simulink model "ADIA"  (R2018b)
settings: Solver=FixedStepDiscrete  StartTime=0.0  StopTime=10.0  FixedStep=0.02  RelTol=1e-3
undefined symbols (not defined in the file or in its folder): ACC_State_Active, ACC_State_BrakeOnly, ACC_State_Suspended, ACC_State_WaitingRise, ADAS_AEBBrakingProg, ADAS_DeclControlReq, ADAS_DriveOff, ADAS_ESCHoldReq_NotHold, ADASDecType_ACC, ADASDecType_AEB, ADIA_ACC_Acceleration_OOR_DecCount_C, ADIA_ACC_Acceleration_OOR_Duration_C, ADIA_ACC_Acceleration_OOR_IncCount_C, ADIA_ACC_Acceleration_OOR_LLim_C, ADIA_ACC_Acceleration_OOR_ULim_C, ADIA_ACC_AccelTrqReq_MixedDia_ULim_C, ADIA_ACC_AccelTrqReq_ULim_C, ADIA_ACC_Deceleration_Mixed_ULim_C, ADIA_ACC_Deceleration_OOR_DecCount_C, ADIA_ACC_Deceleration_OOR_Duration_C, ADIA_ACC_Deceleration_OOR_IncCount_C, ADIA_ACC_Deceleration_OOR_LLim_C, ADIA_ACC_Deceleration_OOR_ULim_C, ADIA_ACC_DriveOff_Distance_C, ADIA_ACC_DriveOff_TimeLim_C, ADIA_ACC_ReqMixed_DecCount_C, ADIA_ACC_ReqMixed_Duration_C, ADIA_ACC_ReqMixed_IncCount_C, ADIA_AccPedalRaw_MaxLim_C, ADIA_AccPedalRaw_MinLim_C, ADIA_ADAS_HoldDecReq_Set_C, ADIA_ADAS_HoldRConfirm_TimeLim_C, ADIA_ADAS_HoldVehSpd_Lim_C, ADIA_AEB_VehSpdDec_LLim_C, ADIA_AEB_VehSpdDec_ULim_C, ADIA_ASWFault_OvrdEn_C, ADIA_ASWFault_OvrdValue_C, ADIA_BatteryOutOfRange_DecCount_C, ADIA_BatteryOutOfRange_Duration_C, ADIA_BatteryOutOfRange_IncCount_C, ADIA_BattVolt_MaxLim_C, ADIA_BattVolt_MinLim_C, ADIA_BCM3_33C_InvBrkLight_DecCount_C, ADIA_BCM3_33C_InvBrkLight_Duration_C, ADIA_BCM3_33C_InvBrkLight_IncCount_C, ADIA_BCM_BattVolt_OvrdEn_C, ADIA_BCM_BattVolt_OvrdVal_C, ADIA_BCM_BrakeLampStaus_OvrdEn_C, ADIA_BCM_BrakeLampStaus_OvrdVal_C, ADIA_BCM_CHMSLStaus_OvrdEn_C, ADIA_BCM_CHMSLStaus_OvrdVal_C, ADIA_BCM_LeftTurnSwSt_OvrdEn_C, ADIA_BCM_LeftTurnSwSt_OvrdVal_C, ADIA_BCM_RightTurnSwSt_OvrdEn_C, ADIA_BCM_RightTurnSwSt_OvrdVal_C, ADIA_BCM_TurnSwFailure_DecCount_C, ADIA_BCM_TurnSwFailure_Duration_C, ADIA_BCM_TurnSwFailure_IncCount_C, ADIA_BSWFault_Ignore_C, ADIA_BSWFault_OvrdEn_C ... (+281)
libraries: simulink x208
(part 10 of 10)

== system ADIA/ADAS_Diagnostics/Diagnostics_Processing/Rationality_Diagnostics/SAS_A5_InvRotSpeed/Counter&Latch/Timer1 ==
  incrcondition : Inport
  incrvalue : Inport  Port=2
  decrcondition : Inport  Port=3
  decvalue : Inport  Port=4
  maxlimit : Inport  Port=5
  reset : Inport  Port=6
  Constant{,1..3} (4 alike) : Constant  Value=0  OutDataTypeStr=Inherit: Inherit via back propagation
  MinMax1 : MinMax  Inputs=2  OutDataTypeStr=Inherit: Inherit via back propagation  InputSameDT=on
  MinMax2 : MinMax  Function=max  Inputs=2  OutDataTypeStr=Inherit: Inherit via back propagation  InputSameDT=on
  Relational Operator : RelationalOperator  OutDataTypeStr=boolean  RndMeth=Nearest
  Sum : Sum  Inputs=++-  OutDataTypeStr=Inherit: Inherit via back propagation  InputSameDT=on
  Unit Delay : UnitDelay  SampleTime=-1
  dec switch : Switch  Criteria=u2 ~= 0  Threshold=1  OutDataTypeStr=Inherit: Inherit via back propagation  InputSameDT=on
  inc switch : Switch  Criteria=u2 ~= 0  Threshold=1  OutDataTypeStr=Inherit: Inherit via back propagation  InputSameDT=on
  reset switch : Switch  Criteria=u2 ~= 0  Threshold=1  OutDataTypeStr=Inherit: Inherit via back propagation  InputSameDT=on
  counter out : Outport
  counter_status : Outport  Port=2
  wires:
  decvalue/1 -> dec switch/1
  Relational Operator/1 -> counter_status/1
  Constant3/1 -> reset switch/1
  inc switch/1 -> Sum/2
  Sum/1 -> MinMax2/2
  maxlimit/1 -> MinMax1/2, Relational Operator/2
  Constant2/1 -> MinMax2/1
  reset switch/1 -> counter out/1, Relational Operator/1, Unit Delay/1
  Unit Delay/1 -> Sum/1
  reset/1 -> reset switch/2
  Constant/1 -> inc switch/3
  MinMax2/1 -> MinMax1/1
  incrvalue/1 -> inc switch/1
  MinMax1/1 -> reset switch/3
  dec switch/1 -> Sum/3
  Constant1/1 -> dec switch/3
  decrcondition/1 -> dec switch/2
  incrcondition/1 -> inc switch/2

== system ADIA/ADAS_Diagnostics/Diagnostics_Processing/Rationality_Diagnostics/SCC_309_OorACCButton/Counter&Latch/Latch  ==
  Input : Inport
  Latch Reset : Inport  Port=2
  Constant11 : Constant  Value=0  OutDataTypeStr=Inherit: Inherit via back propagation
  Constant12 : Constant  OutDataTypeStr=Inherit: Inherit via back propagation
  Switch : Switch  Threshold=1  OutDataTypeStr=Inherit: Inherit via back propagation  SaturateOnIntegerOverflow=on  InputSameDT=on
  Switch1 : Switch  Threshold=1  OutDataTypeStr=Inherit: Inherit via back propagation  SaturateOnIntegerOverflow=on  InputSameDT=on
  Unit Delay1 : UnitDelay  SampleTime=-1
  Output : Outport  InitialOutput=0
  wires:
  Constant12/1 -> Switch1/1
  Constant11/1 -> Switch/1
  Input/1 -> Switch1/2
  Unit Delay1/1 -> Switch1/3
  Switch/1 -> Unit Delay1/1, Output/1
  Latch Reset/1 -> Switch/2
  Switch1/1 -> Switch/3

== system ADIA/ADAS_Diagnostics/Diagnostics_Processing/Rationality_Diagnostics/SCC_309_OorACCButton/Counter&Latch/Timer1 ==
  incrcondition : Inport
  incrvalue : Inport  Port=2
  decrcondition : Inport  Port=3
  decvalue : Inport  Port=4
  maxlimit : Inport  Port=5
  reset : Inport  Port=6
  Constant{,1..3} (4 alike) : Constant  Value=0  OutDataTypeStr=Inherit: Inherit via back propagation
  MinMax1 : MinMax  Inputs=2  OutDataTypeStr=Inherit: Inherit via back propagation  InputSameDT=on
  MinMax2 : MinMax  Function=max  Inputs=2  OutDataTypeStr=Inherit: Inherit via back propagation  InputSameDT=on
  Relational Operator : RelationalOperator  OutDataTypeStr=boolean  RndMeth=Nearest
  Sum : Sum  Inputs=++-  OutDataTypeStr=Inherit: Inherit via back propagation  InputSameDT=on
  Unit Delay : UnitDelay  SampleTime=-1
  dec switch : Switch  Criteria=u2 ~= 0  Threshold=1  OutDataTypeStr=Inherit: Inherit via back propagation  InputSameDT=on
  inc switch : Switch  Criteria=u2 ~= 0  Threshold=1  OutDataTypeStr=Inherit: Inherit via back propagation  InputSameDT=on
  reset switch : Switch  Criteria=u2 ~= 0  Threshold=1  OutDataTypeStr=Inherit: Inherit via back propagation  InputSameDT=on
  counter out : Outport
  counter_status : Outport  Port=2
  wires:
  decvalue/1 -> dec switch/1
  Relational Operator/1 -> counter_status/1
  Constant3/1 -> reset switch/1
  inc switch/1 -> Sum/2
  Sum/1 -> MinMax2/2
  maxlimit/1 -> MinMax1/2, Relational Operator/2
  Constant2/1 -> MinMax2/1
  reset switch/1 -> counter out/1, Relational Operator/1, Unit Delay/1
  Unit Delay/1 -> Sum/1
  reset/1 -> reset switch/2
  Constant/1 -> inc switch/3
  MinMax2/1 -> MinMax1/1
  incrvalue/1 -> inc switch/1
  MinMax1/1 -> reset switch/3
  dec switch/1 -> Sum/3
  Constant1/1 -> dec switch/3
  decrcondition/1 -> dec switch/2
  incrcondition/1 -> inc switch/2

== system ADIA/ADAS_Diagnostics/Diagnostics_Processing/Rationality_Diagnostics/Subsystem1/Counter&Latch/Latch  ==
  Input : Inport
  Latch Reset : Inport  Port=2
  Constant11 : Constant  Value=0  OutDataTypeStr=Inherit: Inherit via back propagation
  Constant12 : Constant  OutDataTypeStr=Inherit: Inherit via back propagation
  Switch : Switch  Threshold=1  OutDataTypeStr=Inherit: Inherit via back propagation  SaturateOnIntegerOverflow=on  InputSameDT=on
  Switch1 : Switch  Threshold=1  OutDataTypeStr=Inherit: Inherit via back propagation  SaturateOnIntegerOverflow=on  InputSameDT=on
  Unit Delay1 : UnitDelay  SampleTime=-1
  Output : Outport  InitialOutput=0
  wires:
  Constant12/1 -> Switch1/1
  Constant11/1 -> Switch/1
  Input/1 -> Switch1/2
  Unit Delay1/1 -> Switch1/3
  Switch/1 -> Unit Delay1/1, Output/1
  Latch Reset/1 -> Switch/2
  Switch1/1 -> Switch/3

== system ADIA/ADAS_Diagnostics/Diagnostics_Processing/Rationality_Diagnostics/Subsystem1/Counter&Latch/Timer1 ==
  incrcondition : Inport
  incrvalue : Inport  Port=2
  decrcondition : Inport  Port=3
  decvalue : Inport  Port=4
  maxlimit : Inport  Port=5
  reset : Inport  Port=6
  Constant{,1..3} (4 alike) : Constant  Value=0  OutDataTypeStr=Inherit: Inherit via back propagation
  MinMax1 : MinMax  Inputs=2  OutDataTypeStr=Inherit: Inherit via back propagation  InputSameDT=on
  MinMax2 : MinMax  Function=max  Inputs=2  OutDataTypeStr=Inherit: Inherit via back propagation  InputSameDT=on
  Relational Operator : RelationalOperator  OutDataTypeStr=boolean  RndMeth=Nearest
  Sum : Sum  Inputs=++-  OutDataTypeStr=Inherit: Inherit via back propagation  InputSameDT=on
  Unit Delay : UnitDelay  SampleTime=-1
  dec switch : Switch  Criteria=u2 ~= 0  Threshold=1  OutDataTypeStr=Inherit: Inherit via back propagation  InputSameDT=on
  inc switch : Switch  Criteria=u2 ~= 0  Threshold=1  OutDataTypeStr=Inherit: Inherit via back propagation  InputSameDT=on
  reset switch : Switch  Criteria=u2 ~= 0  Threshold=1  OutDataTypeStr=Inherit: Inherit via back propagation  InputSameDT=on
  counter out : Outport
  counter_status : Outport  Port=2
  wires:
  decvalue/1 -> dec switch/1
  Relational Operator/1 -> counter_status/1
  Constant3/1 -> reset switch/1
  inc switch/1 -> Sum/2
  Sum/1 -> MinMax2/2
  maxlimit/1 -> MinMax1/2, Relational Operator/2
  Constant2/1 -> MinMax2/1
  reset switch/1 -> counter out/1, Relational Operator/1, Unit Delay/1
  Unit Delay/1 -> Sum/1
  reset/1 -> reset switch/2
  Constant/1 -> inc switch/3
  MinMax2/1 -> MinMax1/1
  incrvalue/1 -> inc switch/1
  MinMax1/1 -> reset switch/3
  dec switch/1 -> Sum/3
  Constant1/1 -> dec switch/3
  decrcondition/1 -> dec switch/2
  incrcondition/1 -> inc switch/2

== system ADIA/ADAS_Diagnostics/Diagnostics_Processing/Rationality_Diagnostics/Subsystem2/Counter&Latch/Latch  ==
  Input : Inport
  Latch Reset : Inport  Port=2
  Constant11 : Constant  Value=0  OutDataTypeStr=Inherit: Inherit via back propagation
  Constant12 : Constant  OutDataTypeStr=Inherit: Inherit via back propagation
  Switch : Switch  Threshold=1  OutDataTypeStr=Inherit: Inherit via back propagation  SaturateOnIntegerOverflow=on  InputSameDT=on
  Switch1 : Switch  Threshold=1  OutDataTypeStr=Inherit: Inherit via back propagation  SaturateOnIntegerOverflow=on  InputSameDT=on
  Unit Delay1 : UnitDelay  SampleTime=-1
  Output : Outport  InitialOutput=0
  wires:
  Constant12/1 -> Switch1/1
  Constant11/1 -> Switch/1
  Input/1 -> Switch1/2
  Unit Delay1/1 -> Switch1/3
  Switch/1 -> Unit Delay1/1, Output/1
  Latch Reset/1 -> Switch/2
  Switch1/1 -> Switch/3

== system ADIA/ADAS_Diagnostics/Diagnostics_Processing/Rationality_Diagnostics/Subsystem2/Counter&Latch/Timer1 ==
  incrcondition : Inport
  incrvalue : Inport  Port=2
  decrcondition : Inport  Port=3
  decvalue : Inport  Port=4
  maxlimit : Inport  Port=5
  reset : Inport  Port=6
  Constant{,1..3} (4 alike) : Constant  Value=0  OutDataTypeStr=Inherit: Inherit via back propagation
  MinMax1 : MinMax  Inputs=2  OutDataTypeStr=Inherit: Inherit via back propagation  InputSameDT=on
  MinMax2 : MinMax  Function=max  Inputs=2  OutDataTypeStr=Inherit: Inherit via back propagation  InputSameDT=on
  Relational Operator : RelationalOperator  OutDataTypeStr=boolean  RndMeth=Nearest
  Sum : Sum  Inputs=++-  OutDataTypeStr=Inherit: Inherit via back propagation  InputSameDT=on
  Unit Delay : UnitDelay  SampleTime=-1
  dec switch : Switch  Criteria=u2 ~= 0  Threshold=1  OutDataTypeStr=Inherit: Inherit via back propagation  InputSameDT=on
  inc switch : Switch  Criteria=u2 ~= 0  Threshold=1  OutDataTypeStr=Inherit: Inherit via back propagation  InputSameDT=on
  reset switch : Switch  Criteria=u2 ~= 0  Threshold=1  OutDataTypeStr=Inherit: Inherit via back propagation  InputSameDT=on
  counter out : Outport
  counter_status : Outport  Port=2
  wires:
  decvalue/1 -> dec switch/1
  Relational Operator/1 -> counter_status/1
  Constant3/1 -> reset switch/1
  inc switch/1 -> Sum/2
  Sum/1 -> MinMax2/2
  maxlimit/1 -> MinMax1/2, Relational Operator/2
  Constant2/1 -> MinMax2/1
  reset switch/1 -> counter out/1, Relational Operator/1, Unit Delay/1
  Unit Delay/1 -> Sum/1
  reset/1 -> reset switch/2
  Constant/1 -> inc switch/3
  MinMax2/1 -> MinMax1/1
  incrvalue/1 -> inc switch/1
  MinMax1/1 -> reset switch/3
  dec switch/1 -> Sum/3
  Constant1/1 -> dec switch/3
  decrcondition/1 -> dec switch/2
  incrcondition/1 -> inc switch/2

== system ADIA/ADAS_Diagnostics/Diagnostics_Processing/Rationality_Diagnostics/Subsystem3/Counter&Latch/Latch  ==
  Input : Inport
  Latch Reset : Inport  Port=2
  Constant11 : Constant  Value=0  OutDataTypeStr=Inherit: Inherit via back propagation
  Constant12 : Constant  OutDataTypeStr=Inherit: Inherit via back propagation
  Switch : Switch  Threshold=1  OutDataTypeStr=Inherit: Inherit via back propagation  SaturateOnIntegerOverflow=on  InputSameDT=on
  Switch1 : Switch  Threshold=1  OutDataTypeStr=Inherit: Inherit via back propagation  SaturateOnIntegerOverflow=on  InputSameDT=on
  Unit Delay1 : UnitDelay  SampleTime=-1
  Output : Outport  InitialOutput=0
  wires:
  Constant12/1 -> Switch1/1
  Constant11/1 -> Switch/1
  Input/1 -> Switch1/2
  Unit Delay1/1 -> Switch1/3
  Switch/1 -> Unit Delay1/1, Output/1
  Latch Reset/1 -> Switch/2
  Switch1/1 -> Switch/3

== system ADIA/ADAS_Diagnostics/Diagnostics_Processing/Rationality_Diagnostics/Subsystem3/Counter&Latch/Timer1 ==
  incrcondition : Inport
  incrvalue : Inport  Port=2
  decrcondition : Inport  Port=3
  decvalue : Inport  Port=4
  maxlimit : Inport  Port=5
  reset : Inport  Port=6
  Constant{,1..3} (4 alike) : Constant  Value=0  OutDataTypeStr=Inherit: Inherit via back propagation
  MinMax1 : MinMax  Inputs=2  OutDataTypeStr=Inherit: Inherit via back propagation  InputSameDT=on
  MinMax2 : MinMax  Function=max  Inputs=2  OutDataTypeStr=Inherit: Inherit via back propagation  InputSameDT=on
  Relational Operator : RelationalOperator  OutDataTypeStr=boolean  RndMeth=Nearest
  Sum : Sum  Inputs=++-  OutDataTypeStr=Inherit: Inherit via back propagation  InputSameDT=on
  Unit Delay : UnitDelay  SampleTime=-1
  dec switch : Switch  Criteria=u2 ~= 0  Threshold=1  OutDataTypeStr=Inherit: Inherit via back propagation  InputSameDT=on
  inc switch : Switch  Criteria=u2 ~= 0  Threshold=1  OutDataTypeStr=Inherit: Inherit via back propagation  InputSameDT=on
  reset switch : Switch  Criteria=u2 ~= 0  Threshold=1  OutDataTypeStr=Inherit: Inherit via back propagation  InputSameDT=on
  counter out : Outport
  counter_status : Outport  Port=2
  wires:
  decvalue/1 -> dec switch/1
  Relational Operator/1 -> counter_status/1
  Constant3/1 -> reset switch/1
  inc switch/1 -> Sum/2
  Sum/1 -> MinMax2/2
  maxlimit/1 -> MinMax1/2, Relational Operator/2
  Constant2/1 -> MinMax2/1
  reset switch/1 -> counter out/1, Relational Operator/1, Unit Delay/1
  Unit Delay/1 -> Sum/1
  reset/1 -> reset switch/2
  Constant/1 -> inc switch/3
  MinMax2/1 -> MinMax1/1
  incrvalue/1 -> inc switch/1
  MinMax1/1 -> reset switch/3
  dec switch/1 -> Sum/3
  Constant1/1 -> dec switch/3
  decrcondition/1 -> dec switch/2
  incrcondition/1 -> inc switch/2

== system ADIA/ADAS_Diagnostics/Diagnostics_Processing/Rationality_Diagnostics/TCU1_93_InvOorGear/Counter&Latch/Latch  ==
  Input : Inport
  Latch Reset : Inport  Port=2
  Constant11 : Constant  Value=0  OutDataTypeStr=Inherit: Inherit via back propagation
  Constant12 : Constant  OutDataTypeStr=Inherit: Inherit via back propagation
  Switch : Switch  Threshold=1  OutDataTypeStr=Inherit: Inherit via back propagation  SaturateOnIntegerOverflow=on  InputSameDT=on
  Switch1 : Switch  Threshold=1  OutDataTypeStr=Inherit: Inherit via back propagation  SaturateOnIntegerOverflow=on  InputSameDT=on
  Unit Delay1 : UnitDelay  SampleTime=-1
  Output : Outport  InitialOutput=0
  wires:
  Constant12/1 -> Switch1/1
  Constant11/1 -> Switch/1
  Input/1 -> Switch1/2
  Unit Delay1/1 -> Switch1/3
  Switch/1 -> Unit Delay1/1, Output/1
  Latch Reset/1 -> Switch/2
  Switch1/1 -> Switch/3

== system ADIA/ADAS_Diagnostics/Diagnostics_Processing/Rationality_Diagnostics/TCU1_93_InvOorGear/Counter&Latch/Timer1 ==
  incrcondition : Inport
  incrvalue : Inport  Port=2
  decrcondition : Inport  Port=3
  decvalue : Inport  Port=4
  maxlimit : Inport  Port=5
  reset : Inport  Port=6
  Constant{,1..3} (4 alike) : Constant  Value=0  OutDataTypeStr=Inherit: Inherit via back propagation
  MinMax1 : MinMax  Inputs=2  OutDataTypeStr=Inherit: Inherit via back propagation  InputSameDT=on
  MinMax2 : MinMax  Function=max  Inputs=2  OutDataTypeStr=Inherit: Inherit via back propagation  InputSameDT=on
  Relational Operator : RelationalOperator  OutDataTypeStr=boolean  RndMeth=Nearest
  Sum : Sum  Inputs=++-  OutDataTypeStr=Inherit: Inherit via back propagation  InputSameDT=on
  Unit Delay : UnitDelay  SampleTime=-1
  dec switch : Switch  Criteria=u2 ~= 0  Threshold=1  OutDataTypeStr=Inherit: Inherit via back propagation  InputSameDT=on
  inc switch : Switch  Criteria=u2 ~= 0  Threshold=1  OutDataTypeStr=Inherit: Inherit via back propagation  InputSameDT=on
  reset switch : Switch  Criteria=u2 ~= 0  Threshold=1  OutDataTypeStr=Inherit: Inherit via back propagation  InputSameDT=on
  counter out : Outport
  counter_status : Outport  Port=2
  wires:
  decvalue/1 -> dec switch/1
  Relational Operator/1 -> counter_status/1
  Constant3/1 -> reset switch/1
  inc switch/1 -> Sum/2
  Sum/1 -> MinMax2/2
  maxlimit/1 -> MinMax1/2, Relational Operator/2
  Constant2/1 -> MinMax2/1
  reset switch/1 -> counter out/1, Relational Operator/1, Unit Delay/1
  Unit Delay/1 -> Sum/1
  reset/1 -> reset switch/2
  Constant/1 -> inc switch/3
  MinMax2/1 -> MinMax1/1
  incrvalue/1 -> inc switch/1
  MinMax1/1 -> reset switch/3
  dec switch/1 -> Sum/3
  Constant1/1 -> dec switch/3
  decrcondition/1 -> dec switch/2
  incrcondition/1 -> inc switch/2

== stateflow chart ADIA/ADAS_Diagnostics/Processing ==
  (default) -> (junction 19)
  (junction 19) -> (junction 6) : {GetData;}
  (junction 6) -> (junction 7) [order 1] : [Diag_Trigger==1]
      | {Process;
      | Output;}
  (junction 6) -> (junction 23) [order 2] : [Diag_Trigger==0]
      | {Timer = Timer +dT}
  (junction 23) -> (junction 7) [order 2]
  (junction 23) -> (junction 7) [order 1] : [(Timer >= DelayTime)==1]
      | {Diag_Trigger=1}
  data: dT input single [0..60]; DelayTime input single; Timer output single [0..60] =0; Diag_Trigger output boolean =0
  events: GetData output FUNCTION_CALL_EVENT; Process output FUNCTION_CALL_EVENT; Output output FUNCTION_CALL_EVENT
